simulink library "PCMULib"  (R2022b)
settings: Solver=ode45  StartTime=0.0  StopTime=10.0  RelTol=1e-3  EnableMultiTasking=on
undefined symbols (not defined in the file or in its folder): BreakpointData, BreakpointData1, BreakpointData2, BreakpointData_One_A, BreakpointData_Two_A, caaaa_dbi, caaaa_swi, cTmComprCtrl_n_i16SM4CmpHeatKiMax, cTmComprCtrl_n_i16SM4CmpHeatKiMin, cTmComprCtrl_n_i16SM4CmpHeatKpMax, cTmComprCtrl_n_i16SM4CmpHeatKpMin, cTmComprCtrl_Te_s32ErrCmpPIContinueHeatH, cTmComprCtrl_Te_s32ErrCmpPIContinueHeatL, cTmIn_n_ElacCmprReq_db, cTmIn_n_ElacCmprReq_sw, db, dbi, E2E_P01DataIDMode, E2E_P01ReceiverStatusType, EnumClass, iBit, initalValue, No_Runnable_Period, ObB_EidBsgStDerat_C, p_OVERRIDE_MASTER_SWITCH, SlDemoSign, sw, swi, SwitchOff_P, SwitchOn_P, Table, TableData_M, VCCTi33, VSysD_FidVehDerat1_C
libraries: simulink x22, CCMLib x11, simulink_need_slupdate x9, UXFD_Lib x7, canmsglib x2, PTCC_Lib x1, hdlsllib x1
(part 5 of 7)

== system PCMULib/Autosar/E2E_P01Protect/E2E_P01Protect ==
  DataLength : Inport
  DataID : Inport  Port=2
  Vmc_Out_BrkActrCtrlModForMinTqReq : Inport  Port=3
  Vmc_Out_BrkTqGrdtNegMinReq : Inport  Port=4
  Vmc_Out_BrkTqGrdtPosMinReq : Inport  Port=5
  Vmc_Out_BrkTqMinReq : Inport  Port=6
  RollingCounter_In : Inport  Port=7
  CheckSum_In : Inport  Port=8
  BusCreator1 : BusCreator  Inputs=1  OutDataTypeStr=Bus: E2E_P01SenderStateType  NonVirtualBus=on
      settings: CopyFcn=set_param(gcbh,'ShowName','off');  InheritFromInputs=off
  BusSelector : BusSelector  OutputSignals=Counter
      settings: CopyFcn=set_param(gcbh,'ShowName','off');
  Data Type Conversion : DataTypeConversion  SaturateOnIntegerOverflow=off  RndMeth=Floor
  Data_Pack : Subsystem
  E2E_Config : Subsystem
  E2E_P01Protect_S : Subsystem
      mask Display:
      | disp('E2E_P01Protect');
      | port_label('input',1,'ConfigType');
      | port_label('input',2,'SenderStateType');
      | port_label('input',3,'Data_pu8');
      | port_label('output',1,'Std_ReturnType');
  Unit Delay : UnitDelay  SampleTime=-1  HasFrameUpgradeWarning=on
  E2E_P01Protect_ReturnType : Outport
  Data_pu8 : Outport  Port=2
  wires:
  BusSelector/1 -> Unit Delay/1  "<Counter>"
  BusCreator1/1 -> E2E_P01Protect_S/2(SenderStateType), BusSelector/1
  Unit Delay/1 -> BusCreator1/1
  E2E_P01Protect_S/1(Std_ReturnType) -> E2E_P01Protect_ReturnType/1
  E2E_Config/1(E2E_P01_Config) -> E2E_P01Protect_S/1(ConfigType)
  DataLength/1 -> E2E_Config/1(DataLength)
  DataID/1 -> E2E_Config/2(DataID)
  Data Type Conversion/1 -> Data_pu8/1, E2E_P01Protect_S/3(Data_pu8)
  Data_Pack/1(Data_pu8) -> Data Type Conversion/1
  Vmc_Out_BrkTqGrdtPosMinReq/1 -> Data_Pack/3(Vmc_Out_BrkTqGrdtPosMinReq)
  Vmc_Out_BrkTqGrdtNegMinReq/1 -> Data_Pack/2(Vmc_Out_BrkTqGrdtNegMinReq)
  Vmc_Out_BrkTqMinReq/1 -> Data_Pack/4(Vmc_Out_BrkTqMinReq)
  Vmc_Out_BrkActrCtrlModForMinTqReq/1 -> Data_Pack/1(Vmc_Out_BrkActrCtrlModForMinTqReq)
  RollingCounter_In/1 -> Data_Pack/5(RollingCounter_In)
  CheckSum_In/1 -> Data_Pack/6(CheckSum_In)

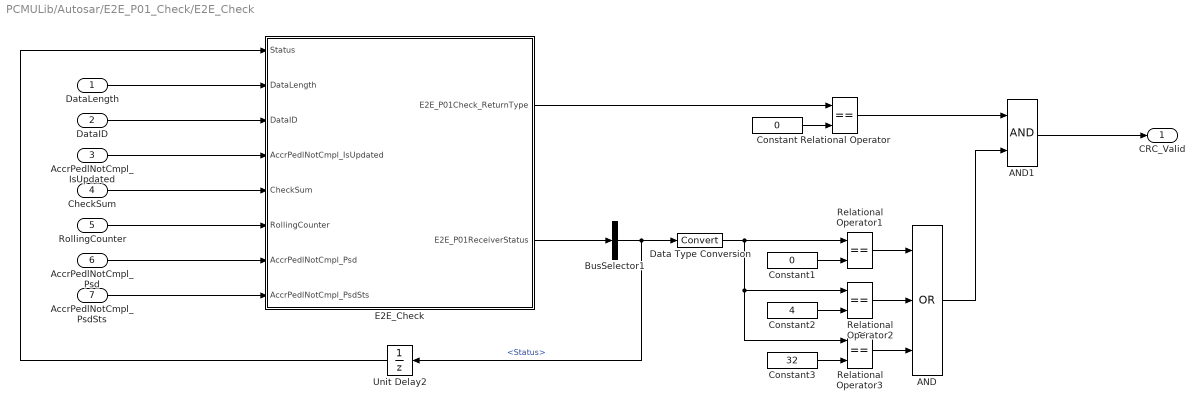
== system PCMULib/Autosar/E2E_P01_Check/E2E_Check ==
  DataLength : Inport
  DataID : Inport  Port=2
  AccrPedlNotCmpl_IsUpdated : Inport  Port=3
  CheckSum : Inport  Port=4
  RollingCounter : Inport  Port=5
  AccrPedlNotCmpl_Psd : Inport  Port=6
  AccrPedlNotCmpl_PsdSts : Inport  Port=7
  AND : Logic  Operator=OR  Inputs=3  AllPortsSameDT=off  OutDataTypeStr=boolean
      settings: CopyFcn=set_param(gcbh,'ShowName','off');
  AND1 : Logic  AllPortsSameDT=off  OutDataTypeStr=boolean
      settings: CopyFcn=set_param(gcbh,'ShowName','off');
  BusSelector1 : BusSelector  OutputSignals=Status
      settings: CopyFcn=set_param(gcbh,'ShowName','off');
  Constant : Constant  Value=0  OutDataTypeStr=Inherit: Inherit via back propagation
      settings: CopyFcn=set_param(gcbh,'ShowName','off');
  Constant1 : Constant  Value=0  OutDataTypeStr=Inherit: Inherit via back propagation
      settings: CopyFcn=set_param(gcbh,'ShowName','off');
  Constant2 : Constant  Value=4  OutDataTypeStr=Inherit: Inherit via back propagation
      settings: CopyFcn=set_param(gcbh,'ShowName','off');
  Constant3 : Constant  Value=32  OutDataTypeStr=Inherit: Inherit via back propagation
      settings: CopyFcn=set_param(gcbh,'ShowName','off');
  Data Type Conversion : DataTypeConversion  SaturateOnIntegerOverflow=off  RndMeth=Floor
  E2E_Check : Subsystem  TreatAsAtomicUnit=on
  Relational Operator{,1..3} (4 alike) : RelationalOperator  Operator===  OutDataTypeStr=boolean  InputSameDT=off
      settings: CopyFcn=set_param(gcbh,'ShowName','off');
  Unit Delay2 : UnitDelay  InitialCondition=E2E_P01ReceiverStatusType.E2E_P01STATUS_OK  SampleTime=-1  HasFrameUpgradeWarning=on
  CRC_Valid : Outport
  wires:
  BusSelector1/1 -> Data Type Conversion/1, Unit Delay2/1  "<Status>"
  DataLength/1 -> E2E_Check/2(DataLength)
  DataID/1 -> E2E_Check/3(DataID)
  AccrPedlNotCmpl_IsUpdated/1 -> E2E_Check/4(AccrPedlNotCmpl_IsUpdated)
  CheckSum/1 -> E2E_Check/5(CheckSum)
  RollingCounter/1 -> E2E_Check/6(RollingCounter)
  Unit Delay2/1 -> E2E_Check/1(Status)
  E2E_Check/1(E2E_P01Check_ReturnType) -> Relational Operator/1
  E2E_Check/2(E2E_P01ReceiverStatus) -> BusSelector1/1
  Constant/1 -> Relational Operator/2
  Constant1/1 -> Relational Operator1/2
  Constant2/1 -> Relational Operator2/2
  Constant3/1 -> Relational Operator3/2
  Relational Operator1/1 -> AND/1
  Relational Operator3/1 -> AND/3
  Relational Operator2/1 -> AND/2
  AND1/1 -> CRC_Valid/1
  Data Type Conversion/1 -> Relational Operator3/1, Relational Operator2/1, Relational Operator1/1
  AccrPedlNotCmpl_Psd/1 -> E2E_Check/7(AccrPedlNotCmpl_Psd)
  AccrPedlNotCmpl_PsdSts/1 -> E2E_Check/8(AccrPedlNotCmpl_PsdSts)
  Relational Operator/1 -> AND1/1
  AND/1 -> AND1/2

== system PCMULib/CCM/LowPass filter Resettable/Unit Delay Resettable External IC boolean controlled ==
  u : Inport  OutDataTypeStr=dt
  R : Inport  Port=2  OutDataTypeStr=boolean
  IC : Inport  Port=3  OutDataTypeStr=dt
  FixPt Constant : Constant  DisableCoverage=on  Value=false  OutDataTypeStr=boolean  SampleTime=-1
  FixPt Data Type Duplicate1 : DataTypeDuplicate  DisableCoverage=on  NumInputPorts=4
  FixPt Logical Operator : Logic  DisableCoverage=on  Operator=OR  AllPortsSameDT=off  OutDataTypeStr=boolean
  FixPt Unit Delay1 : UnitDelay  DisableCoverage=on  InitialCondition=UnitDelayInitCondition  SampleTime=-1
  FixPt Unit Delay2 : UnitDelay  DisableCoverage=on  InitialCondition=true  SampleTime=-1  HasFrameUpgradeWarning=on
  Init : Switch  Criteria=u2 ~= 0  OutDataTypeStr=Inherit: Inherit via back propagation  ZeroCross=off  InputSameDT=off
  Reset : Switch  Criteria=u2 ~= 0  OutDataTypeStr=Inherit: Inherit via back propagation  ZeroCross=off  InputSameDT=off
  y : Outport  OutDataTypeStr=dt
  wires:
  FixPt Logical Operator/1 -> Init/2
  FixPt Unit Delay1/1 -> Init/3
  Init/1 -> y/1, FixPt Data Type Duplicate1/1
  FixPt Unit Delay2/1 -> FixPt Logical Operator/2
  FixPt Constant/1 -> FixPt Unit Delay2/1
  R/1 -> FixPt Logical Operator/1, Reset/2
  Reset/1 -> FixPt Unit Delay1/1, FixPt Data Type Duplicate1/2
  u/1 -> Reset/3, FixPt Data Type Duplicate1/4
  IC/1 -> FixPt Data Type Duplicate1/3, Init/1, Reset/1

== system PCMULib/CCM/LowPass filter IC Resettable/Unit Delay Resettable External IC boolean controlled ==
  u : Inport  OutDataTypeStr=dt
  R : Inport  Port=2  OutDataTypeStr=boolean
  IC : Inport  Port=3  OutDataTypeStr=dt
  FixPt Constant : Constant  DisableCoverage=on  Value=false  OutDataTypeStr=boolean  SampleTime=-1
  FixPt Data Type Duplicate1 : DataTypeDuplicate  DisableCoverage=on  NumInputPorts=4
  FixPt Logical Operator : Logic  DisableCoverage=on  Operator=OR  AllPortsSameDT=off  OutDataTypeStr=boolean
  FixPt Unit Delay1 : UnitDelay  DisableCoverage=on  InitialCondition=UnitDelayInitCondition  SampleTime=-1
  FixPt Unit Delay2 : UnitDelay  DisableCoverage=on  InitialCondition=true  SampleTime=-1  HasFrameUpgradeWarning=on
  Init : Switch  Criteria=u2 ~= 0  OutDataTypeStr=Inherit: Inherit via back propagation  ZeroCross=off  InputSameDT=off
  Reset : Switch  Criteria=u2 ~= 0  OutDataTypeStr=Inherit: Inherit via back propagation  ZeroCross=off  InputSameDT=off
  y : Outport  OutDataTypeStr=dt
  wires:
  IC/1 -> Reset/1, Init/1, FixPt Data Type Duplicate1/3
  u/1 -> FixPt Data Type Duplicate1/4, Reset/3
  Reset/1 -> FixPt Data Type Duplicate1/2, FixPt Unit Delay1/1
  R/1 -> Reset/2, FixPt Logical Operator/1
  FixPt Constant/1 -> FixPt Unit Delay2/1
  FixPt Unit Delay2/1 -> FixPt Logical Operator/2
  Init/1 -> FixPt Data Type Duplicate1/1, y/1
  FixPt Unit Delay1/1 -> Init/3
  FixPt Logical Operator/1 -> Init/2

== system PCMULib/CCM/Rate Limiter Resettable IC/Unit Delay Resettable External IC boolean controlled ==
  u : Inport  OutDataTypeStr=dt
  R : Inport  Port=2  OutDataTypeStr=boolean
  IC : Inport  Port=3  OutDataTypeStr=dt
  FixPt Constant : Constant  DisableCoverage=on  Value=false  OutDataTypeStr=boolean  SampleTime=-1
  FixPt Data Type Duplicate1 : DataTypeDuplicate  DisableCoverage=on  NumInputPorts=4
  FixPt Logical Operator : Logic  DisableCoverage=on  Operator=OR  AllPortsSameDT=off  OutDataTypeStr=boolean
  FixPt Unit Delay1 : UnitDelay  DisableCoverage=on  InitialCondition=UnitDelayInitCondition  SampleTime=-1
  FixPt Unit Delay2 : UnitDelay  DisableCoverage=on  InitialCondition=true  SampleTime=-1  HasFrameUpgradeWarning=on
  Init : Switch  Criteria=u2 ~= 0  OutDataTypeStr=Inherit: Inherit via back propagation  ZeroCross=off  InputSameDT=off
  Reset : Switch  Criteria=u2 ~= 0  OutDataTypeStr=Inherit: Inherit via back propagation  ZeroCross=off  InputSameDT=off
  y : Outport  OutDataTypeStr=dt
  wires:
  FixPt Logical Operator/1 -> Init/2
  FixPt Unit Delay1/1 -> Init/3
  Init/1 -> y/1, FixPt Data Type Duplicate1/1
  FixPt Unit Delay2/1 -> FixPt Logical Operator/2
  FixPt Constant/1 -> FixPt Unit Delay2/1
  R/1 -> FixPt Logical Operator/1, Reset/2
  Reset/1 -> FixPt Unit Delay1/1, FixPt Data Type Duplicate1/2
  u/1 -> Reset/3, FixPt Data Type Duplicate1/4
  IC/1 -> FixPt Data Type Duplicate1/3, Init/1, Reset/1

== system PCMULib/Calculation/PI/PID_Saturation ==
  note: 0=Not saturated
      | 1=Saturated TOP
      | 2=SaturatedBottom
      | 3=Saturated both (?!?)
  up : Inport
  u : Inport  Port=2
  lo : Inport  Port=3
  Data Type Duplicate : DataTypeDuplicate
  Data Type Propagation : simulink/Signal Attributes/Data Type Propagation  PropDataType=fixdt('double')  IfRefDouble=double  IfRefSingle=single  IsSigned=IsSigned1  NumBitsBase=NumBits1  NumBitsMult=1  NumBitsAdd=0  NumBitsAllowFinal=1:128  PropScaling=[]  ValuesUsedBestPrec=[5 -7]  SlopeBase=Slope1  SlopeMult=1  SlopeAdd=0  BiasBase=Bias1  BiasMult=1  BiasAdd=0
  Gain : Gain  Gain=2  ParamDataTypeStr=uint8  OutDataTypeStr=uint8
  HitLowerLimit : RelationalOperator  DisableCoverage=on  Operator=<  OutDataTypeStr=boolean  InputSameDT=off
  HitUpperLimit : RelationalOperator  DisableCoverage=on  Operator=>  OutDataTypeStr=boolean  InputSameDT=off
  Sum : Sum  Inputs=+|+  AccumDataTypeStr=uint8  OutDataTypeStr=uint8
  Switch : Switch  Criteria=u2 ~= 0  OutDataTypeStr=Inherit: Inherit via back propagation  RndMeth=Nearest  ZeroCross=off  InputSameDT=off
  Switch2 : Switch  Criteria=u2 ~= 0  OutMin=OutMin  OutMax=OutMax  RndMeth=Nearest  ZeroCross=off  InputSameDT=off
  y : Outport  OutMin=OutMin  OutMax=OutMax  VectorParamsAs1DForOutWhenUnconnected=off
  N_SaturationState : Outport  Port=2  OutMin=OutMin  OutMax=OutMax  OutDataTypeStr=uint8  VectorParamsAs1DForOutWhenUnconnected=off
  wires:
  HitLowerLimit/1 -> Switch/2, Gain/1
  HitUpperLimit/1 -> Switch2/2, Sum/1
  Switch2/1 -> y/1, Data Type Duplicate/1
  Switch/1 -> Data Type Propagation/3, Switch2/3, Data Type Duplicate/2
  lo/1 -> HitLowerLimit/2, Switch/1
  u/1 -> HitLowerLimit/1, Switch/3, HitUpperLimit/1, Data Type Propagation/1, Data Type Propagation/2
  up/1 -> HitUpperLimit/2, Switch2/1
  Gain/1 -> Sum/2
  Sum/1 -> N_SaturationState/1

== system PCMULib/Calculation/PI/SaturationAndDeadband ==
  note: 1) 当前压缩机目标转速小于等于压缩机最低限制时:
      | A. 如果Er ≤ cTmComprCtrl_Te_s32ErrCmpPIContinueHeatL，跳过PI 计算；
      | B. 如果Er > 0，PI 继续运算；
      | 2) 当前压缩机目标转速大于等于压缩机最高限制时：
      | A. 如果Er ≥ cTmComprCtrl_Te_s32ErrCmpPIContinueHeatH，跳过PI 计算；
      | B. 如果Er < 0，PI 继续运算；
  note: 2=SaturatedBottom
  note: 3=Saturated both (UL=LL)
  note: 1=Saturated TOP
  note: 0=Not saturated
  Error : Inport
  Deadband : Inport  Port=2
  N_SaturationState : Inport  Port=3  OutDataTypeStr=uint8
  Constant : Constant  Value=0  OutDataTypeStr=Inherit: Inherit via back propagation  SampleTime=-1
  Constant1 : Constant  Value=0  OutDataTypeStr=Inherit: Inherit via back propagation  SampleTime=-1
  DB : Switch  Criteria=u2 ~= 0  Threshold=0.5
  ErrorLargerThanDeadband : RelationalOperator  Operator=>  OutDataTypeStr=boolean  ZeroCross=off
  Multiport Switch : MultiPortSwitch  DataPortOrder=Zero-based contiguous  Inputs=4  zeroidx=on  SaturateOnIntegerOverflow=off  InputSameDT=off
  Relay1 : Relay  OnSwitchValue=0  OffSwitchValue=cTmComprCtrl_Te_s32ErrCmpPIContinueHeatL  OutDataTypeStr=boolean
  Relay3 : Relay  OnSwitchValue=cTmComprCtrl_Te_s32ErrCmpPIContinueHeatH  OffSwitchValue=0  OnOutputValue=0  OffOutputValue=1  OutDataTypeStr=boolean
  Switch : Switch  Criteria=u2 > Threshold  SaturateOnIntegerOverflow=off  InputSameDT=off
  Switch1 : Switch  Criteria=u2 > Threshold  SaturateOnIntegerOverflow=off  InputSameDT=off
  absolute : Subsystem
  Error Out : Outport  VectorParamsAs1DForOutWhenUnconnected=off
  wires:
  DB/1 -> Multiport Switch/5, Switch1/1, Relay1/1, Switch/1, Relay3/1, Multiport Switch/2
  absolute/1(Output) -> ErrorLargerThanDeadband/1
  ErrorLargerThanDeadband/1 -> DB/2
  N_SaturationState/1 -> Multiport Switch/1
  Switch/1 -> Multiport Switch/4
  Switch1/1 -> Multiport Switch/3
  Multiport Switch/1 -> Error Out/1
  Constant/1 -> DB/3
  Deadband/1 -> ErrorLargerThanDeadband/2
  Error/1 -> DB/1, absolute/1(Input)
  Relay3/1 -> Switch/2
  Constant1/1 -> Switch1/3, Switch/3
  Relay1/1 -> Switch1/2

== system PCMULib/Custom/CAN/CAN_Receive ==
  In1 : Inport
  In2 : Inport  Port=2
  Return_Value : S-Function  FunctionName=ACTION_CANBSW_RecMsg_S  SFunctionDeploymentMode=off  EnableBusSupport=off
  Out1 : Outport
  wires:
  Return_Value/1 -> Out1/1
  In2/1 -> Return_Value/2
  In1/1 -> Return_Value/1

== system PCMULib/Custom/CAN/CAN_Transmit ==
  In1 : Inport
  In2 : Inport  Port=2
  S-Function : S-Function  FunctionName=ACTION_CANBSW_SndMsg_S  SFunctionDeploymentMode=off  EnableBusSupport=off
  Out1 : Outport
  wires:
  In1/1 -> S-Function/1
  In2/1 -> S-Function/2
  S-Function/1 -> Out1/1

== system PCMULib/Custom/CAN/CanHex2Signed ==
  note: 计算判断条件： 2 n-1 -1
      | 和2^n
  note: 判断输入的BitLength是否（0<u1<=32bit）;
      | 并向下取整。
  hex : Inport
  Add4 : Sum
      settings: CopyFcn=set_param(gcbh,'ShowName','off');
  Constant1 : Constant  Value=BitLength
  Constant5 : Constant  Value=Factor
  Constant6 : Constant  Value=Offset
  If : If  IfExpression=u1 == 1
      settings: CopyFcn=set_param(gcbh,'ShowName','off');
  Merge : Merge
      settings: CopyFcn=set_param(gcbh,'ShowName','off');
  Product : Product  OutDataTypeStr=single
      settings: CopyFcn=set_param(gcbh,'ShowName','off');
  Relational Operator : RelationalOperator  Operator=<  OutDataTypeStr=boolean  InputSameDT=off
  condtion : Subsystem
  signal_conditioning : Subsystem
  value<0 : Subsystem  TreatAsAtomicUnit=on
  value>0 : Subsystem  TreatAsAtomicUnit=on
  Out1 : Outport
  wires:
  value>0/1(Out1) -> Merge/2
  [index] -> value<0/2(2^n)
  condtion/2(2^n) -> [index]
  Relational Operator/1 -> If/1
  If/1 -> value<0/Action
  If/2 -> value>0/Action
  hex/1 -> Relational Operator/2, value<0/1(hex), value>0/1(hex)
  condtion/1(cond) -> Relational Operator/1
  signal_conditioning/1(BitLength_BeUsed) -> condtion/1(bitL)
  Constant6/1 -> Add4/2
  Add4/1 -> Out1/1
  Merge/1 -> Product/1
  Product/1 -> Add4/1
  Constant5/1 -> Product/2
  value<0/1(Out1) -> Merge/1
  Constant1/1 -> signal_conditioning/1(In1)

== system PCMULib/Custom/CAN/Get_MsgLength ==
  In1 : Inport
  msg_length : S-Function  FunctionName=msg_length_s  SFunctionDeploymentMode=off  EnableBusSupport=off
  Out1 : Outport
  wires:
  msg_length/1 -> Out1/1
  In1/1 -> msg_length/1

== system PCMULib/Custom/CAN/xbackground1 ==

== system PCMULib/Custom/Diagnose/Dem_SetEventStatus ==
  EveSt : Inport
  bEna : Inport  Port=2
  DEM_EventID : Constant  Value=EventID  SampleTime=-1
  Dem_SetEventStatus_Enable : Subsystem
  wires:
  bEna/1 -> Dem_SetEventStatus_Enable/Enable
  EveSt/1 -> Dem_SetEventStatus_Enable/2(EveSt)
  DEM_EventID/1 -> Dem_SetEventStatus_Enable/1(EventID)

== system PCMULib/Custom/Diagnose/Fim_GetFunctionPermission ==
  FIM_EventID : Constant  Value=FunctionID  SampleTime=-1
  Fim_GetFunctionPermission_Asw : S-Function  FunctionName=Fim_GetFunctionPermission_Asw_SF  SFunctionDeploymentMode=off  EnableBusSupport=off  mask(Legacy Function){SFunctionSpec=void Fim_GetFunctionPermission_Asw(uint16 u1, boolean y1[1]), ShowSpec=on}
      mask prompts: ShowSpec "Display function specification"
      mask help:
      | This block allows you to call the legacy functions specified by the following Legacy Code Tool definition:
      | def.SFunctionName = 'Fim_GetFunctionPermission_Asw_SF';
      | def.OutputFcnSpec = 'void Fim_GetFunctionPermission_Asw(uint16 u1, boolean y1[1])';
      | def.HeaderFiles = {'Fim.h'};
      | def.SourceFiles = {'Fim.c'};
      mask Help: <p>This block was generated automatically by the Legacy Code Tool. For detailed help on this tool, call<a href="matlab:legacy_code('help')"> legacy_code('help')</a>.</p>
      mask Callback ShowSpec:
      | if strcmp(get_param(gcbh, 'ShowSpec'), 'on')
      |   set_param(gcbh, 'MaskDisplay', sprintf('fprintf(''%s'');', get_param(gcbh, 'SFunctionSpec')));
      | else
      |   set_param(gcbh, 'MaskDisplay', sprintf('fprintf(''%s'');', get_param(gcbh, 'FunctionName')));
      | end
      mask Display: fprintf('void Fim_GetFunctionPermission_Asw(uint16 u1, boolean y1[1])');
  bPermission : Outport
  wires:
  Fim_GetFunctionPermission_Asw/1 -> bPermission/1
  FIM_EventID/1 -> Fim_GetFunctionPermission_Asw/1

== system PCMULib/Custom/Diagnose/xbackground1 ==

== system PCMULib/Custom/PIN/PIN ADC ==
  Enable : EnablePort
  S-Function : S-Function  FunctionName=Sws_Io_Adc_Get_xxx_S  SFunctionDeploymentMode=off  EnableBusSupport=off
  Value : Outport
  wires:
  S-Function/1 -> Value/1

== system PCMULib/Custom/PIN/PIN DI ==
  Enable : EnablePort
  S-Function : S-Function  FunctionName=Sws_Io_Dio_Get_xxx_S  SFunctionDeploymentMode=off  EnableBusSupport=off
  Value : Outport
  wires:
  S-Function/1 -> Value/1

== system PCMULib/Custom/PIN/PIN DO ==
  In1 : Inport  OutDataTypeStr=boolean
  Enable : EnablePort
  S-Function : S-Function  FunctionName=Sws_Io_Dio_Set_O_S_xxx_S  SFunctionDeploymentMode=off  EnableBusSupport=off
  wires:
  In1/1 -> S-Function/1

== system PCMULib/Custom/PIN/PIN DO1 ==
  In1 : Inport  OutDataTypeStr=int16
  In2 : Inport  Port=2  OutDataTypeStr=uint32
  Enable : EnablePort
  S-Function : S-Function  FunctionName=Sws_Io_Pwm_SetPeriodAndDuty_xxx_S  SFunctionDeploymentMode=off  EnableBusSupport=off
  wires:
  In1/1 -> S-Function/1
  In2/1 -> S-Function/2

== system PCMULib/Custom/PIN/PIN ICU ==
  Enable : EnablePort
  S-Function : S-Function  FunctionName=Sws_Io_Icu_GetDutyCycle_xxx_S  SFunctionDeploymentMode=off  EnableBusSupport=off
  Value : Outport
  wires:
  S-Function/1 -> Value/1

== system PCMULib/Custom/PIN/xbackground1 ==

== system PCMULib/Standard/Bit Operation/GetBitFnc ==
  BitVal : Inport  OutDataTypeStr=uint32
  Bitwise Operator4 : simulink/Logic and Bit Operations/Bitwise Operator  logicop=AND  UseBitMask=off  NumInputPorts=2  BitMask=bin2dec('1111111111111111')  BitMaskRealWorld=Real World Value
  Data Type Conversion2 : DataTypeConversion  SaturateOnIntegerOverflow=off  RndMeth=Floor
  Fcn : Fcn  Expr=2^u
  Getbit_n : Constant  Value=uint8(2)  OutDataTypeStr=single  SampleTime=-1
  Max : Constant  Value=uint8(31)  OutDataTypeStr=single  SampleTime=-1
  Min : Constant  Value=uint8(0)  OutDataTypeStr=single  SampleTime=-1
  Saturation : UXFD_Lib/Standard/Math/Saturation
  Shift Arithmetic4 : ArithShift  BitShiftNumber=GetBitPar  BitShiftDirection=Right
  Out1 : Outport
  wires:
  Bitwise Operator4/1 -> Shift Arithmetic4/1
  Shift Arithmetic4/1 -> Out1/1
  Saturation/1 -> Fcn/1
  Max/1 -> Saturation/2
  Min/1 -> Saturation/3
  BitVal/1 -> Bitwise Operator4/1
  Fcn/1 -> Data Type Conversion2/1
  Getbit_n/1 -> Saturation/1
  Data Type Conversion2/1 -> Bitwise Operator4/2

== system PCMULib/Standard/Bit Operation/SetBitFnc ==
  BitVal : Inport  OutDataTypeStr=boolean
  BitWise : simulink/Logic and Bit Operations/Bitwise Operator  logicop=AND  UseBitMask=on  BitMask=bin2dec('11111111111111111111111111111111')  BitMaskRealWorld=Stored Integer
  Data Type Conversion : DataTypeConversion  SaturateOnIntegerOverflow=off  RndMeth=Floor
  Data Type Conversion1 : DataTypeConversion  RndMeth=Simplest  SaturateOnIntegerOverflow=off
  Fcn : Fcn  Expr=2^u
  Max : Constant  Value=uint8(31)  OutDataTypeStr=single  SampleTime=-1
  Min : Constant  Value=uint8(0)  OutDataTypeStr=single  SampleTime=-1
  Product : Product  OutDataTypeStr=uint32
      settings: CopyFcn=set_param(gcbh,'ShowName','off');
  Saturation : UXFD_Lib/Standard/Math/Saturation
  Setbit_n : Constant  Value=uint8(5)  OutDataTypeStr=single  SampleTime=-1
  Out : Outport
  wires:
  BitVal/1 -> Data Type Conversion1/1
  BitWise/1 -> Out/1
  Product/1 -> BitWise/1
  Setbit_n/1 -> Saturation/1
  Fcn/1 -> Data Type Conversion/1
  Data Type Conversion/1 -> Product/2
  Data Type Conversion1/1 -> Product/1
  Saturation/1 -> Fcn/1
  Max/1 -> Saturation/2
  Min/1 -> Saturation/3

== system PCMULib/Standard/Calibration/1-D Lookup Table Without Const_Param ==
  note: Lookup Table 1D ( AVLib™ )
  u : Inport  OutDataTypeStr=double
  Curve : Lookup  InputValues=BreakpointData  Table=Table  LookUpMeth=Interpolation-Use End Values  OutDataTypeStr=double  SaturateOnIntegerOverflow=off
  y : Outport  OutMin=OutMin  OutMax=OutMax
  wires:
  Curve/1 -> y/1
  u/1 -> Curve/1

== system PCMULib/Standard/Calibration/2-D Lookup Table Without Const_Param ==
  note: Lookup Table 2D ( AVLib™ )
  u1 : Inport  OutDataTypeStr=double
  u2 : Inport  Port=2  OutDataTypeStr=double
  Map : Lookup2D  RowIndex=BreakpointData1  ColumnIndex=BreakpointData2  Table=Table  LookUpMeth=Interpolation-Use End Values  OutDataTypeStr=double  SaturateOnIntegerOverflow=off  InputSameDT=off
  y : Outport  OutMin=OutMin  OutMax=OutMax
  wires:
  Map/1 -> y/1
  u2/1 -> Map/2
  u1/1 -> Map/1

== system PCMULib/Standard/Calibration/OverRide ==
  override_value : Inport
  switch : Inport  Port=2
  input : Inport  Port=3
  Data Type Conversion2 : DataTypeConversion  OutDataTypeStr=boolean  SaturateOnIntegerOverflow=off  RndMeth=Floor
  Switch1 : Switch  Criteria=u2 ~= 0  Threshold=1  RndMeth=Zero  SaturateOnIntegerOverflow=off
      settings: AttributesFormatString=%<Criteria>
  Out : Outport
  wires:
  Data Type Conversion2/1 -> Switch1/2
  override_value/1 -> Switch1/1
  switch/1 -> Data Type Conversion2/1
  Switch1/1 -> Out/1
  input/1 -> Switch1/3

== system PCMULib/Standard/Calibration/OverRide_with_master_switch ==
  override_value : Inport
  switch : Inport  Port=2
  input : Inport  Port=3
  Constant : Constant  Value=p_OVERRIDE_MASTER_SWITCH
  Constant1 : Constant  Value=85  OutDataTypeStr=uint8
  Data Type Conversion2 : DataTypeConversion  OutDataTypeStr=boolean  SaturateOnIntegerOverflow=off  RndMeth=Floor
  Logical Operator : Logic
  Relational Operator1 : RelationalOperator  Operator===  OutDataTypeStr=boolean
  Switch1 : Switch  Criteria=u2 ~= 0  Threshold=1  RndMeth=Zero  SaturateOnIntegerOverflow=off
      settings: AttributesFormatString=%<Criteria>
  Out : Outport
  wires:
  Constant1/1 -> Relational Operator1/2
  Relational Operator1/1 -> Logical Operator/2
  input/1 -> Switch1/3
  Switch1/1 -> Out/1
  override_value/1 -> Switch1/1
  Data Type Conversion2/1 -> Switch1/2
  switch/1 -> Logical Operator/1
  Logical Operator/1 -> Data Type Conversion2/1
  Constant/1 -> Relational Operator1/1

== system PCMULib/Standard/Calibration/xbackground1 ==

== system PCMULib/Standard/Calibration/xbackground2 ==

== system PCMULib/Standard/Calibration/xbackground3 ==

== system PCMULib/Standard/Calibration/xbackground4 ==

== system PCMULib/Standard/Discrete dynamics/BumplessRateTransfer ==
  s : Inport
  u1 : Inport  Port=2
  u0 : Inport  Port=3
  d10 : Inport  Port=4
  d01 : Inport  Port=5
  Add : Sum  Inputs=-+
  Add1 : Sum
  Constant1 : Constant  Value=0
  Constant2 : Constant
  LogicalSwitch1 : Subsystem  mask(GL_LogicSwitch_1.0){}
      mask init:
      | set_param(gcb,'LinkStatus','none');
      mask Display:
      | plot([-0.1 0.2 0.2], [0.85 0.85 0.75])
      | plot([-0.1 0.2 0.2], [0.5 0.5 0.6])
      | plot([0.8 1.1], [0.5 0.5])
      | plot([0.15 0.8], [0.6 0.5])
      | plot([-0.1 0.5 0.5], [0.15 0.15 0.6])
  Product : Product
  RateLimit : Subsystem  mask(PAG_Rate_Limiter_LV1.1_BV2){}
      mask help:
      | Rate limiter.
      | Limits the derivative of the input signal to a
      | value beween df (fall rate) and dr (rise rate).
      mask Display:
      | plot([0.35, 0.55, 0.55, 1.0], [0, 0, 1, 1])
      | plot([0.35, 0.55, 0.8, 1.0], [0, 0, 1, 1])
  Tq_EngInstReq_ : Outport
  wires:
  Add/1 -> Product/1
  Product/1 -> Add1/2
  Add1/1 -> Tq_EngInstReq_/1
  u0/1 -> Add1/1, Add/1
  u1/1 -> Add/2
  s/1 -> LogicalSwitch1/3(In3)
  Constant2/1 -> LogicalSwitch1/1(In1)
  Constant1/1 -> LogicalSwitch1/2(In2)
  d10/1 -> RateLimit/3(df)
  d01/1 -> RateLimit/2(dr)
  LogicalSwitch1/1(Out1) -> RateLimit/1(In1)
  RateLimit/1(y) -> Product/2

== system PCMULib/Standard/Discrete dynamics/BumplessTransfer ==
  s : Inport
  u1 : Inport  Port=2
  u0 : Inport  Port=3
  tc : Inport  Port=4
  Add : Sum  Inputs=-+
  Add1 : Sum
  Constant : Constant  Value=0  OutDataTypeStr=Inherit: Inherit via back propagation
  Constant1 : Constant  OutDataTypeStr=Inherit: Inherit via back propagation
  LPF1_pole1 : Subsystem  mask(PAG_FirstOrder_Lowpass_Filter_LV1.1_BV2){}
      mask help:
      | Discrete low-pass filter. Corresponding analogue transfer function:
      |   1 / (1 + tau * s)
      mask Display:
      | plot([0.35, 0.9], [0, 0], [0.35, 0.35], [0, 1])
      | plot(0.35:0.55/10:0.9,   [0 0.39 0.63 0.78 0.86 0.92 0.95 0.98 0.99 0.99 0.99])
  LogicalSwitch1 : Subsystem  mask(GL_LogicSwitch_1.0){}
      mask init:
      | set_param(gcb,'LinkStatus','none');
      mask Display:
      | plot([-0.1 0.2 0.2], [0.85 0.85 0.75])
      | plot([-0.1 0.2 0.2], [0.5 0.5 0.6])
      | plot([0.8 1.1], [0.5 0.5])
      | plot([0.15 0.8], [0.6 0.5])
      | plot([-0.1 0.5 0.5], [0.15 0.15 0.6])
  Product : Product
  Out : Outport
  wires:
  Add/1 -> Product/1
  u0/1 -> Add1/1, Add/1
  s/1 -> LogicalSwitch1/3(In3)
  Product/1 -> Add1/2
  Add1/1 -> Out/1
  u1/1 -> Add/2
  LogicalSwitch1/1(Out1) -> LPF1_pole1/1(u)
  Constant1/1 -> LogicalSwitch1/1(In1)
  Constant/1 -> LogicalSwitch1/2(In2)
  LPF1_pole1/1(y) -> Product/2
  tc/1 -> LPF1_pole1/2(tc)

== system PCMULib/Standard/Discrete dynamics/DLPF1_pole_v2 ==
  u : Inport
  tc : Inport  Port=2
  Add : Sum
  Add1 : Sum  Inputs=-+
  Add2 : Sum
  Add3 : Sum  Inputs=+-
  Constant : Constant  Value=0
  Constant1 : Constant  Value=0
  Constant2 : Constant  Value=1e-6
  Constant3 : Constant  Value=1e-6
  Divide : Product  Inputs=*/
  Divide1 : Product  Inputs=*/
  LogicalSwitch1 : Subsystem  mask(GL_LogicSwitch_1.0){}
      mask init:
      | set_param(gcb,'LinkStatus','none');
      mask Display:
      | plot([-0.1 0.2 0.2], [0.85 0.85 0.75])
      | plot([-0.1 0.2 0.2], [0.5 0.5 0.6])
      | plot([0.8 1.1], [0.5 0.5])
      | plot([0.15 0.8], [0.6 0.5])
      | plot([-0.1 0.5 0.5], [0.15 0.15 0.6])
  MinMax : MinMax  Function=max  Inputs=2
  MinMax1 : MinMax  Function=max  Inputs=2
  Product : Product
  Unit Delay : UnitDelay  SampleTime=-1  HasFrameUpgradeWarning=on
  Unit Delay1 : UnitDelay  SampleTime=-1  HasFrameUpgradeWarning=on
  Unit Delay2 : UnitDelay  SampleTime=-1  HasFrameUpgradeWarning=on
  ts : DataStoreRead  DataStoreName=ts  IndexOptions=Index vector (dialog)  Indices=1  OutputSizes=1
  y : Outport
  wires:
  tc/1 -> Add2/2
  MinMax1/1 -> Divide/2
  Constant3/1 -> MinMax1/2
  Add2/1 -> MinMax1/1
  u/1 -> Add3/1, Unit Delay/1
  Unit Delay/1 -> Add3/2
  Add3/1 -> Divide1/1
  Product/1 -> Add/2
  Divide1/1 -> Add1/2
  Unit Delay1/1 -> Add1/1, Add/1
  Divide/1 -> Product/2
  Add1/1 -> Product/1
  MinMax/1 -> Divide1/2
  Constant2/1 -> MinMax/2
  ts/1 -> Add2/1, MinMax/1, Divide/1
  Unit Delay2/1 -> LogicalSwitch1/3(In3)
  Constant1/1 -> Unit Delay2/1
  Constant/1 -> LogicalSwitch1/1(In1)
  Add/1 -> LogicalSwitch1/2(In2)
  LogicalSwitch1/1(Out1) -> Unit Delay1/1, y/1

== system PCMULib/Standard/Discrete dynamics/FirstOrderFilter ==
  u : Inport
  tc : Inport  Port=2
  Constant1 : Constant  Value=1e-6  OutDataTypeStr=single  mask(TL_Constant){data={'output',{'type','Float32'},'date',735300.29228814819}}
      settings: CopyFcn=if exist('tl_reset_reviewflag','file')==2,tl_reset_reviewflag(gcbh);end  DeleteFcn=if exist('delete_tlblock','file')==2,delete_tlblock(gcbh);end  NameChangeFcn=if exist('rename_tlblock','file')==2,rename_tlblock(gcbh);end  OpenFcn=if exist('tl_open_blockdlg','file')==2,tl_open_blockdlg(gcbh);else,open_system(gcbh,'parameter');end
      mask Help: eval(['if exist(''tl_online_help'',''file'') == 2, tl_online_help(''Topic'',''TL_Constant''),else, web([''jar:file:///'',matlabroot,''/help/toolbox/simulink/help.jar!/slref/' lower(get_param(gcbh,'Blocktype')) '.html''], ''-helpbrowser''),end'])
      mask Display: plot([-0.05, 1.05, NaN, -0.05, 1.05],[.01, .01, NaN, .99, .99])
  Del1 : UnitDelay  SampleTime=-1  HasFrameUpgradeWarning=on  mask(TL_UnitDelay){data={'logdata',{'maxnumvals',4096,'plotchannels',[]},'output',{'type','Float32'},'state',{'type','Float32'},'date',735300.29228789348}}
      settings: CopyFcn=if exist('tl_reset_reviewflag','file')==2,tl_reset_reviewflag(gcbh);end  DeleteFcn=if exist('delete_tlblock','file')==2,delete_tlblock(gcbh);end  NameChangeFcn=if exist('rename_tlblock','file')==2,rename_tlblock(gcbh);end  OpenFcn=if exist('tl_open_blockdlg','file')==2,tl_open_blockdlg(gcbh);else,open_system(gcbh,'parameter');end
      mask Help: eval(['if exist(''tl_online_help'',''file'') == 2, tl_online_help(''Topic'',''TL_UnitDelay''),else, web([''jar:file:///'',matlabroot,''/help/toolbox/simulink/help.jar!/slref/' lower(get_param(gcbh,'Blocktype')) '.html''], ''-helpbrowser''),end'])
      mask Display: plot([-0.05, 1.05, NaN, -0.05, 1.05],[.01, .01, NaN, .99, .99])
  MinMax : MinMax  Function=max  Inputs=3  InputSameDT=on  mask(TL_MinMax){data={'logdata',{'maxnumvals',4096,'plotchannels',[]},'output',{'type','Float32'},'date',735300.29228754633}}
      settings: CopyFcn=if exist('tl_reset_reviewflag','file')==2,tl_reset_reviewflag(gcbh);end  DeleteFcn=if exist('delete_tlblock','file')==2,delete_tlblock(gcbh);end  NameChangeFcn=if exist('rename_tlblock','file')==2,rename_tlblock(gcbh);end  OpenFcn=if exist('tl_open_blockdlg','file')==2,tl_open_blockdlg(gcbh);else,open_system(gcbh,'parameter');end
      mask Help: eval(['if exist(''tl_online_help'',''file'') == 2, tl_online_help(''Topic'',''TL_MinMax''),else, web([''jar:file:///'',matlabroot,''/help/toolbox/simulink/help.jar!/slref/' lower(get_param(gcbh,'Blocktype')) '.html''], ''-helpbrowser''),end'])
      mask Display: plot([-0.05, 1.05, NaN, -0.05, 1.05],[.01, .01, NaN, .99, .99])
  Prod1 : Product  Inputs=*/  InputSameDT=on  RndMeth=Zero  OutDataTypeStr=Inherit: Same as first input  mask(TL_Product){data={'logdata',{'maxnumvals',4096,'plotchannels',[]},'output',{'type','Float32'},'date',735300.29228725692}}
      settings: CopyFcn=if exist('tl_reset_reviewflag','file')==2,tl_reset_reviewflag(gcbh);end  DeleteFcn=if exist('delete_tlblock','file')==2,delete_tlblock(gcbh);end  NameChangeFcn=if exist('rename_tlblock','file')==2,rename_tlblock(gcbh);end  OpenFcn=if exist('tl_open_blockdlg','file')==2,tl_open_blockdlg(gcbh);else,open_system(gcbh,'parameter');end
      mask Help: eval(['if exist(''tl_online_help'',''file'') == 2, tl_online_help(''Topic'',''TL_Product''),else, web([''jar:file:///'',matlabroot,''/help/toolbox/simulink/help.jar!/slref/' lower(get_param(gcbh,'Blocktype')) '.html''], ''-helpbrowser''),end'])
      mask Display: plot([-0.05, 1.05, NaN, -0.05, 1.05],[.01, .01, NaN, .99, .99])
  Prod2 : Product  InputSameDT=on  RndMeth=Zero  OutDataTypeStr=Inherit: Same as first input  mask(TL_Product){data={'logdata',{'maxnumvals',4096,'plotchannels',[]},'output',{'type','Float32'},'date',735300.29228697915}}
      settings: CopyFcn=if exist('tl_reset_reviewflag','file')==2,tl_reset_reviewflag(gcbh);end  DeleteFcn=if exist('delete_tlblock','file')==2,delete_tlblock(gcbh);end  NameChangeFcn=if exist('rename_tlblock','file')==2,rename_tlblock(gcbh);end  OpenFcn=if exist('tl_open_blockdlg','file')==2,tl_open_blockdlg(gcbh);else,open_system(gcbh,'parameter');end
      mask Help: eval(['if exist(''tl_online_help'',''file'') == 2, tl_online_help(''Topic'',''TL_Product''),else, web([''jar:file:///'',matlabroot,''/help/toolbox/simulink/help.jar!/slref/' lower(get_param(gcbh,'Blocktype')) '.html''], ''-helpbrowser''),end'])
      mask Display: plot([-0.05, 1.05, NaN, -0.05, 1.05],[.01, .01, NaN, .99, .99])
  Sum1 : Sum  Inputs=-+  InputSameDT=on  OutDataTypeStr=Inherit: Same as first input  mask(TL_Sum){data={'logdata',{'maxnumvals',4096,'plotchannels',[]},'output',{'type','Float32'},'date',735300.29228671291}}
      settings: CopyFcn=if exist('tl_reset_reviewflag','file')==2,tl_reset_reviewflag(gcbh);end  DeleteFcn=if exist('delete_tlblock','file')==2,delete_tlblock(gcbh);end  NameChangeFcn=if exist('rename_tlblock','file')==2,rename_tlblock(gcbh);end  OpenFcn=if exist('tl_open_blockdlg','file')==2,tl_open_blockdlg(gcbh);else,open_system(gcbh,'parameter');end
      mask Help: eval(['if exist(''tl_online_help'',''file'') == 2, tl_online_help(''Topic'',''TL_Sum''),else, web([''jar:file:///'',matlabroot,''/help/toolbox/simulink/help.jar!/slref/' lower(get_param(gcbh,'Blocktype')) '.html''], ''-helpbrowser''),end'])
      mask Display: plot([-0.05, 1.05, NaN, -0.05, 1.05],[.01, .01, NaN, .99, .99])
  Sum2 : Sum  InputSameDT=on  OutDataTypeStr=Inherit: Same as first input  mask(TL_Sum){data={'logdata',{'maxnumvals',4096,'plotchannels',[]},'output',{'type','Float32'},'date',735300.29228643514}}
      settings: CopyFcn=if exist('tl_reset_reviewflag','file')==2,tl_reset_reviewflag(gcbh);end  DeleteFcn=if exist('delete_tlblock','file')==2,delete_tlblock(gcbh);end  NameChangeFcn=if exist('rename_tlblock','file')==2,rename_tlblock(gcbh);end  OpenFcn=if exist('tl_open_blockdlg','file')==2,tl_open_blockdlg(gcbh);else,open_system(gcbh,'parameter');end
      mask Help: eval(['if exist(''tl_online_help'',''file'') == 2, tl_online_help(''Topic'',''TL_Sum''),else, web([''jar:file:///'',matlabroot,''/help/toolbox/simulink/help.jar!/slref/' lower(get_param(gcbh,'Blocktype')) '.html''], ''-helpbrowser''),end'])
      mask Display: plot([-0.05, 1.05, NaN, -0.05, 1.05],[.01, .01, NaN, .99, .99])
  ts : DataStoreRead  DataStoreName=ts  IndexOptions=Index vector (dialog)  Indices=1  OutputSizes=1  mask(TL_DataStoreRead){data={'logdata',{'plotchannels',[]},'date',735300.29228620371}}
      settings: AttributesFormatString=ts  DeleteFcn=if exist('delete_tlblock','file')==2,delete_tlblock(gcbh);end  NameChangeFcn=if exist('rename_tlblock','file')==2,rename_tlblock(gcbh);end  OpenFcn=if exist('tl_open_blockdlg','file')==2,tl_open_blockdlg(gcbh);else,open_system(gcbh,'parameter');end
      mask Help: eval(['if exist(''tl_online_help'',''file'') == 2, tl_online_help(''Topic'',''TL_DataStoreRead''),else, web([''jar:file:///'',matlabroot,''/help/toolbox/simulink/help.jar!/slref/' lower(get_param(gcbh,'Blocktype')) '.html''], ''-helpbrowser''),end'])
      mask Display: plot([-0.05, 1.05, NaN, -0.05, 1.05],[.01, .01, NaN, .99, .99])
  y : Outport
  wires:
  u/1 -> Sum1/2
  Sum1/1 -> Prod2/1
  MinMax/1 -> Prod1/2
  ts/1 -> Prod1/1, MinMax/1
  Prod1/1 -> Prod2/2
  Del1/1 -> Sum1/1, Sum2/1
  Sum2/1 -> y/1, Del1/1
  tc/1 -> MinMax/2
  Prod2/1 -> Sum2/2
  Constant1/1 -> MinMax/3

== system PCMULib/Standard/Discrete dynamics/FirstOrderFilter1 ==
  u : Inport
  r : Inport  Port=2
  rv : Inport  Port=3
  tc inc : Inport  Port=4
  tc dec : Inport  Port=5
  Constant : Constant  Value=0  mask(TL_Constant){data={'output',{'type','Float32'},'date',735300.29228606483}}
      settings: CopyFcn=if exist('tl_reset_reviewflag','file')==2,tl_reset_reviewflag(gcbh);end  DeleteFcn=if exist('delete_tlblock','file')==2,delete_tlblock(gcbh);end  NameChangeFcn=if exist('rename_tlblock','file')==2,rename_tlblock(gcbh);end  OpenFcn=if exist('tl_open_blockdlg','file')==2,tl_open_blockdlg(gcbh);else,open_system(gcbh,'parameter');end
      mask Help: eval(['if exist(''tl_online_help'',''file'') == 2, tl_online_help(''Topic'',''TL_Constant''),else, web([''jar:file:///'',matlabroot,''/help/toolbox/simulink/help.jar!/slref/' lower(get_param(gcbh,'Blocktype')) '.html''], ''-helpbrowser''),end'])
      mask Display: plot([-0.05, 1.05, NaN, -0.05, 1.05],[.01, .01, NaN, .99, .99])
  Constant1 : Constant  Value=1e-6  OutDataTypeStr=single  mask(TL_Constant){data={'output',{'type','Float32'},'date',735300.29228582175}}
      settings: CopyFcn=if exist('tl_reset_reviewflag','file')==2,tl_reset_reviewflag(gcbh);end  DeleteFcn=if exist('delete_tlblock','file')==2,delete_tlblock(gcbh);end  NameChangeFcn=if exist('rename_tlblock','file')==2,rename_tlblock(gcbh);end  OpenFcn=if exist('tl_open_blockdlg','file')==2,tl_open_blockdlg(gcbh);else,open_system(gcbh,'parameter');end
      mask Help: eval(['if exist(''tl_online_help'',''file'') == 2, tl_online_help(''Topic'',''TL_Constant''),else, web([''jar:file:///'',matlabroot,''/help/toolbox/simulink/help.jar!/slref/' lower(get_param(gcbh,'Blocktype')) '.html''], ''-helpbrowser''),end'])
      mask Display: plot([-0.05, 1.05, NaN, -0.05, 1.05],[.01, .01, NaN, .99, .99])
  Del1 : UnitDelay  SampleTime=-1  HasFrameUpgradeWarning=on  mask(TL_UnitDelay){data={'logdata',{'maxnumvals',4096,'plotchannels',[]},'output',{'type','Float32'},'state',{'type','Float32'},'date',735300.29228555551}}
      settings: CopyFcn=if exist('tl_reset_reviewflag','file')==2,tl_reset_reviewflag(gcbh);end  DeleteFcn=if exist('delete_tlblock','file')==2,delete_tlblock(gcbh);end  NameChangeFcn=if exist('rename_tlblock','file')==2,rename_tlblock(gcbh);end  OpenFcn=if exist('tl_open_blockdlg','file')==2,tl_open_blockdlg(gcbh);else,open_system(gcbh,'parameter');end
      mask Help: eval(['if exist(''tl_online_help'',''file'') == 2, tl_online_help(''Topic'',''TL_UnitDelay''),else, web([''jar:file:///'',matlabroot,''/help/toolbox/simulink/help.jar!/slref/' lower(get_param(gcbh,'Blocktype')) '.html''], ''-helpbrowser''),end'])
      mask Display: plot([-0.05, 1.05, NaN, -0.05, 1.05],[.01, .01, NaN, .99, .99])
  Demux : Demux  Outputs=2
      settings: DisplayOption=none
  Max2 : MinMax  Function=max  Inputs=2  mask(TL_MinMax){data={'logdata',{'plotchannels',[]},'output',{'type','Float32'},'date',735300.29228521988}}
      settings: CopyFcn=if exist('tl_reset_reviewflag','file')==2,tl_reset_reviewflag(gcbh);end  DeleteFcn=if exist('delete_tlblock','file')==2,delete_tlblock(gcbh);end  NameChangeFcn=if exist('rename_tlblock','file')==2,rename_tlblock(gcbh);end  OpenFcn=if exist('tl_open_blockdlg','file')==2,tl_open_blockdlg(gcbh);else,open_system(gcbh,'parameter');end
      mask Help: eval(['if exist(''tl_online_help'',''file'') == 2, tl_online_help(''Topic'',''TL_MinMax''),else, web([''jar:file:///'',matlabroot,''/help/toolbox/simulink/help.jar!/slref/' lower(get_param(gcbh,'Blocktype')) '.html''], ''-helpbrowser''),end'])
      mask Display: plot([-0.05, 1.05, NaN, -0.05, 1.05],[.01, .01, NaN, .99, .99])
  Min : MinMax  Inputs=2  mask(TL_MinMax){data={'logdata',{'plotchannels',[]},'output',{'type','Float32'},'date',735300.29228494212}}
      settings: CopyFcn=if exist('tl_reset_reviewflag','file')==2,tl_reset_reviewflag(gcbh);end  DeleteFcn=if exist('delete_tlblock','file')==2,delete_tlblock(gcbh);end  NameChangeFcn=if exist('rename_tlblock','file')==2,rename_tlblock(gcbh);end  OpenFcn=if exist('tl_open_blockdlg','file')==2,tl_open_blockdlg(gcbh);else,open_system(gcbh,'parameter');end
      mask Help: eval(['if exist(''tl_online_help'',''file'') == 2, tl_online_help(''Topic'',''TL_MinMax''),else, web([''jar:file:///'',matlabroot,''/help/toolbox/simulink/help.jar!/slref/' lower(get_param(gcbh,'Blocktype')) '.html''], ''-helpbrowser''),end'])
      mask Display: plot([-0.05, 1.05, NaN, -0.05, 1.05],[.01, .01, NaN, .99, .99])
  MinMax : MinMax  Function=max  Inputs=3  InputSameDT=on  mask(TL_MinMax){data={'logdata',{'maxnumvals',4096,'plotchannels',[]},'output',{'type','Float32'},'date',735300.29228465282}}
      settings: CopyFcn=if exist('tl_reset_reviewflag','file')==2,tl_reset_reviewflag(gcbh);end  DeleteFcn=if exist('delete_tlblock','file')==2,delete_tlblock(gcbh);end  NameChangeFcn=if exist('rename_tlblock','file')==2,rename_tlblock(gcbh);end  OpenFcn=if exist('tl_open_blockdlg','file')==2,tl_open_blockdlg(gcbh);else,open_system(gcbh,'parameter');end
      mask Help: eval(['if exist(''tl_online_help'',''file'') == 2, tl_online_help(''Topic'',''TL_MinMax''),else, web([''jar:file:///'',matlabroot,''/help/toolbox/simulink/help.jar!/slref/' lower(get_param(gcbh,'Blocktype')) '.html''], ''-helpbrowser''),end'])
      mask Display: plot([-0.05, 1.05, NaN, -0.05, 1.05],[.01, .01, NaN, .99, .99])
  Mux : Mux  Inputs=2
  Mux1 : Mux  Inputs=2
  Prod1 : Product  Inputs=*/  InputSameDT=on  RndMeth=Zero  OutDataTypeStr=Inherit: Same as first input  mask(TL_Product){data={'logdata',{'maxnumvals',4096,'plotchannels',[]},'output',{'type','Float32'},'date',735300.29228437506}}
      settings: CopyFcn=if exist('tl_reset_reviewflag','file')==2,tl_reset_reviewflag(gcbh);end  DeleteFcn=if exist('delete_tlblock','file')==2,delete_tlblock(gcbh);end  NameChangeFcn=if exist('rename_tlblock','file')==2,rename_tlblock(gcbh);end  OpenFcn=if exist('tl_open_blockdlg','file')==2,tl_open_blockdlg(gcbh);else,open_system(gcbh,'parameter');end
      mask Help: eval(['if exist(''tl_online_help'',''file'') == 2, tl_online_help(''Topic'',''TL_Product''),else, web([''jar:file:///'',matlabroot,''/help/toolbox/simulink/help.jar!/slref/' lower(get_param(gcbh,'Blocktype')) '.html''], ''-helpbrowser''),end'])
      mask Display: plot([-0.05, 1.05, NaN, -0.05, 1.05],[.01, .01, NaN, .99, .99])
  Prod2 : Product  InputSameDT=on  RndMeth=Zero  OutDataTypeStr=Inherit: Same as first input  mask(TL_Product){data={'logdata',{'maxnumvals',4096,'plotchannels',[]},'output',{'type','Float32'},'date',735300.29228409717}}
      settings: CopyFcn=if exist('tl_reset_reviewflag','file')==2,tl_reset_reviewflag(gcbh);end  DeleteFcn=if exist('delete_tlblock','file')==2,delete_tlblock(gcbh);end  NameChangeFcn=if exist('rename_tlblock','file')==2,rename_tlblock(gcbh);end  OpenFcn=if exist('tl_open_blockdlg','file')==2,tl_open_blockdlg(gcbh);else,open_system(gcbh,'parameter');end
      mask Help: eval(['if exist(''tl_online_help'',''file'') == 2, tl_online_help(''Topic'',''TL_Product''),else, web([''jar:file:///'',matlabroot,''/help/toolbox/simulink/help.jar!/slref/' lower(get_param(gcbh,'Blocktype')) '.html''], ''-helpbrowser''),end'])
      mask Display: plot([-0.05, 1.05, NaN, -0.05, 1.05],[.01, .01, NaN, .99, .99])
  Sum1 : Sum  Inputs=-+  InputSameDT=on  OutDataTypeStr=Inherit: Same as first input  mask(TL_Sum){data={'logdata',{'maxnumvals',4096,'plotchannels',[]},'output',{'type','Float32'},'date',735300.29228373838}}
      settings: CopyFcn=if exist('tl_reset_reviewflag','file')==2,tl_reset_reviewflag(gcbh);end  DeleteFcn=if exist('delete_tlblock','file')==2,delete_tlblock(gcbh);end  NameChangeFcn=if exist('rename_tlblock','file')==2,rename_tlblock(gcbh);end  OpenFcn=if exist('tl_open_blockdlg','file')==2,tl_open_blockdlg(gcbh);else,open_system(gcbh,'parameter');end
      mask Help: eval(['if exist(''tl_online_help'',''file'') == 2, tl_online_help(''Topic'',''TL_Sum''),else, web([''jar:file:///'',matlabroot,''/help/toolbox/simulink/help.jar!/slref/' lower(get_param(gcbh,'Blocktype')) '.html''], ''-helpbrowser''),end'])
      mask Display: plot([-0.05, 1.05, NaN, -0.05, 1.05],[.01, .01, NaN, .99, .99])
  Sum2 : Sum  Inputs=+++  InputSameDT=on  OutDataTypeStr=Inherit: Same as first input  mask(TL_Sum){data={'logdata',{'maxnumvals',4096,'plotchannels',[]},'output',{'type','Float32'},'date',735300.29228347226}}
      settings: CopyFcn=if exist('tl_reset_reviewflag','file')==2,tl_reset_reviewflag(gcbh);end  DeleteFcn=if exist('delete_tlblock','file')==2,delete_tlblock(gcbh);end  NameChangeFcn=if exist('rename_tlblock','file')==2,rename_tlblock(gcbh);end  OpenFcn=if exist('tl_open_blockdlg','file')==2,tl_open_blockdlg(gcbh);else,open_system(gcbh,'parameter');end
      mask Help: eval(['if exist(''tl_online_help'',''file'') == 2, tl_online_help(''Topic'',''TL_Sum''),else, web([''jar:file:///'',matlabroot,''/help/toolbox/simulink/help.jar!/slref/' lower(get_param(gcbh,'Blocktype')) '.html''], ''-helpbrowser''),end'])
      mask Display: plot([-0.05, 1.05, NaN, -0.05, 1.05],[.01, .01, NaN, .99, .99])
  Switch : Switch  Criteria=u2 ~= 0  Threshold=0.5  SaturateOnIntegerOverflow=off  InputSameDT=off  mask(TL_Switch){data={'logdata',{'plotchannels',[]},'output',{'type','Float32'},'date',735300.29228318285}}
      settings: CopyFcn=if exist('tl_reset_reviewflag','file')==2,tl_reset_reviewflag(gcbh);end  DeleteFcn=if exist('delete_tlblock','file')==2,delete_tlblock(gcbh);end  NameChangeFcn=if exist('rename_tlblock','file')==2,rename_tlblock(gcbh);end  OpenFcn=if exist('tl_open_blockdlg','file')==2,tl_open_blockdlg(gcbh);else,open_system(gcbh,'parameter');end
      mask Help: eval(['if exist(''tl_online_help'',''file'') == 2, tl_online_help(''Topic'',''TL_Switch''),else, web([''jar:file:///'',matlabroot,''/help/toolbox/simulink/help.jar!/slref/' lower(get_param(gcbh,'Blocktype')) '.html''], ''-helpbrowser''),end'])
      mask Display: plot([-0.05, 1.05, NaN, -0.05, 1.05],[.01, .01, NaN, .99, .99])
  ts : DataStoreRead  DataStoreName=ts  IndexOptions=Index vector (dialog)  Indices=1  OutputSizes=1  mask(TL_DataStoreRead){data={'logdata',{'plotchannels',[]},'date',735300.29228288191}}
      settings: AttributesFormatString=ts  DeleteFcn=if exist('delete_tlblock','file')==2,delete_tlblock(gcbh);end  NameChangeFcn=if exist('rename_tlblock','file')==2,rename_tlblock(gcbh);end  OpenFcn=if exist('tl_open_blockdlg','file')==2,tl_open_blockdlg(gcbh);else,open_system(gcbh,'parameter');end
      mask Help: eval(['if exist(''tl_online_help'',''file'') == 2, tl_online_help(''Topic'',''TL_DataStoreRead''),else, web([''jar:file:///'',matlabroot,''/help/toolbox/simulink/help.jar!/slref/' lower(get_param(gcbh,'Blocktype')) '.html''], ''-helpbrowser''),end'])
      mask Display: plot([-0.05, 1.05, NaN, -0.05, 1.05],[.01, .01, NaN, .99, .99])
  y : Outport
  wires:
  Del1/1 -> Sum2/1, Sum1/1
  Prod1/1 -> Prod2/2
  ts/1 -> Prod1/1, MinMax/1
  MinMax/1 -> Prod1/2
  Sum1/1 -> Prod2/1
  u/1 -> Sum1/2
  tc inc/1 -> Mux/1
  tc dec/1 -> Mux/2
  Constant1/1 -> Mux1/1, Mux1/2
  Prod2/1 -> Demux/1
  Demux/1 -> Max2/1
  Demux/2 -> Min/2
  Constant/1 -> Max2/2, Min/1
  Max2/1 -> Sum2/2
  Min/1 -> Sum2/3
  Sum2/1 -> Switch/3
  rv/1 -> Switch/1
  r/1 -> Switch/2
  Switch/1 -> Del1/1, y/1
  Mux/1 -> MinMax/2
  Mux1/1 -> MinMax/3

== system PCMULib/Standard/Discrete dynamics/HysteresisFilter ==
  note: Filter to avoid occilation during low slipp
      | when converter character is steep
  n_Eng5 : Inport
  n_Eng1 : Inport  Port=2
  Add : Sum
  Add1 : Sum  Inputs=+-
  Saturation1 : Subsystem  mask(GL_Saturation_1.0){}
      mask help:
      | If input_1 > input_2
      |   output = input_2
      | elseif input_1 < input_3
      |   output = input_3
      | else
      |   output = input_1
      |
      | Note that if the lower limit is set above the upper limit, the output will take the value of the input to the lower limit port.
      mask init:
      | set_param(gcb,'LinkStatus','none');
      mask Display: plot([0.3, 0.5, 0.7, 0.9], [0, 0, 1, 1])
  Unit Delay : UnitDelay  SampleTime=-1  HasFrameUpgradeWarning=on
  y : Outport
  wires:
  n_Eng5/1 -> Add/1, Add1/1
  Add1/1 -> Saturation1/3(L)
  Add/1 -> Saturation1/2(U)
  Saturation1/1(y) -> Unit Delay/1, y/1
  Unit Delay/1 -> Saturation1/1(u)
  n_Eng1/1 -> Add/2, Add1/2
